simulink model "CS_ABS_KN_S"  (R2019a)
settings: Solver=ode45  StartTime=0  StopTime=10  FixedStep=0.002  RelTol=1e-6  AbsTol=1e-6
values from neighbouring files (symbols this model uses):
  AdCo = 0    [CS_ABS_KN.m]
  MoInRed = SloInRed/SloIn    (= 0.666666666667)    [CS_ABS_KN.m]
  RBP = 0.4    [CS_ABS_KN.m]
  SlMax = 0.15    [CS_ABS_KN.m]
  SloDe_ = SloDe/MBP    (= 3.33333333333)    [CS_ABS_KN.m]
  SloIn_ = SloIn/MBP    (= 10)    [CS_ABS_KN.m]
undefined symbols (not defined in the file or in its folder): DiscIntNeverNeededParam
libraries: Solver_SF x1
settings Model: ExtModeTrigMode=oneshot  ExtModeArmWhenConnect=off  Creator=Malan  LastModifiedBy=d001896
settings SolverCC: AutoScaleAbsTol=off  AlgebraicLoopSolver=LineSearch
settings DataIOCC: SaveFormat=Array  SignalLoggingSaveFormat=ModelDataLogs  ReturnWorkspaceOutputs=off  SignalLoggingName=sigsOut
settings OptimizationCC: BlockReduction=off  BooleanDataType=off  ExpressionDepthLimit=2147483647  InitFltsAndDblsToZero=on  LifeSpan=inf
settings DebuggingCC: AlgebraicLoopMsg=none  SaveWithParameterizedLinksMsg=none  UnderspecifiedInitializationDetection=Classic  MergeDetectMultiDrivingBlocksExec=none  SignalResolutionControl=TryResolveAllWithWarning  InheritedTsInSrcMsg=none  MultiTaskDSMMsg=warning  MultiTaskCondExecSysMsg=none  FcnCallInpInsideContextMsg=warning  StateNameClashWarn=warning  SFUnexpectedBacktrackingDiag=warning  SFNoUnconditionalDefaultTransitionDiag=warning  SFExecutionAtInitializationDiag=none  ArithmeticOperatorsInVariantConditions=warning
settings HardwareCC: ProdBitPerPointer=32  ProdBitPerSizeT=32  ProdBitPerPtrDiffT=32  ProdLargestAtomicFloat=None  ProdIntDivRoundTo=Undefined  ProdEndianess=Unspecified  ProdWordSize=32  ProdHWDeviceType=32-bit Generic  TargetUnknown=on
settings ModelReferenceCC: PropagateSignalLabelsOutOfModel=off
settings SFSimCC: SimUseLocalCustomCode=off
settings RTWCC: TemplateMakefile=grt_vc.tmf  RTWUseLocalCustomCode=off
settings CodeAppCC: StateflowObjectComments=on
settings GRTTargetCC: TargetFcnLib=ansi_tfl_tmw.mat  TargetLangStandard=C89/C90 (ANSI)  CombineOutputUpdateFcns=off  GRTInterface=on
settings ConfigComp: CovMetricSettings=dw  CovHtmlReporting=on  CovSaveCumulativeToWorkspaceVar=on  CovSaveSingleToWorkspaceVar=on  CovExternalEMLEnable=off

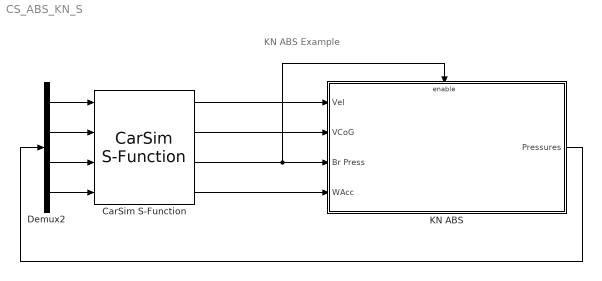
== system CS_ABS_KN_S ==
  note: KN ABS Example
  CarSim S-Function : Solver_SF/CarSim S-Function  Priority=1  SIMFILE=simfile.sim
  Demux2 : Demux
  KN ABS : Subsystem
  wires:
  CarSim S-Function/1 -> KN ABS/1(Vel)
  CarSim S-Function/2 -> KN ABS/2(VCoG)
  CarSim S-Function/3 -> KN ABS/Enable, KN ABS/3(Br Press)
  CarSim S-Function/4 -> KN ABS/4(WAcc)
  KN ABS/1(Pressures) -> Demux2/1
  Demux2/1 -> CarSim S-Function/1
  Demux2/2 -> CarSim S-Function/2
  Demux2/3 -> CarSim S-Function/3
  Demux2/4 -> CarSim S-Function/4

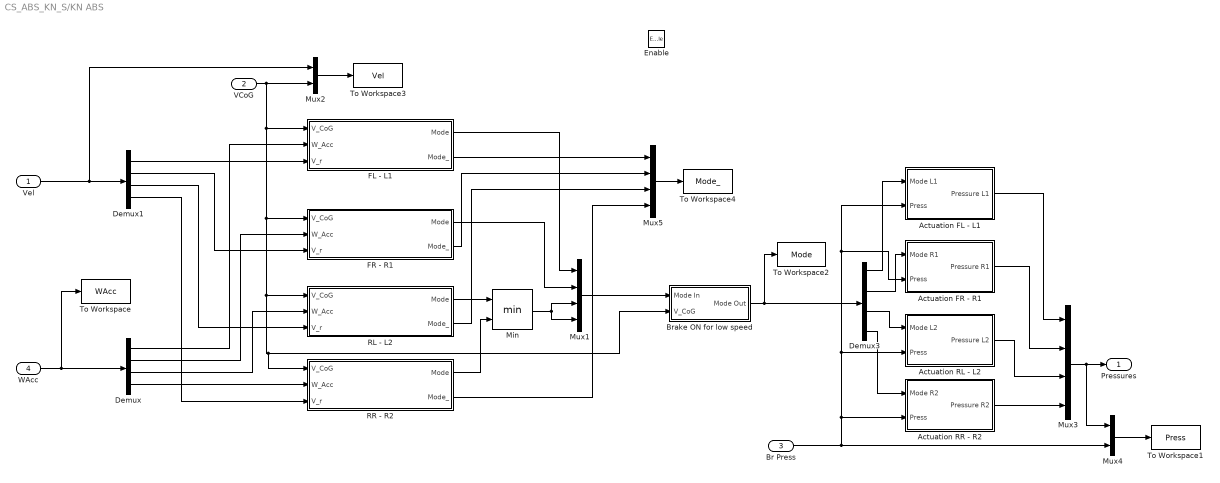
== system CS_ABS_KN_S/KN ABS ==
  Vel : Inport
  VCoG : Inport  Port=2
  Br Press : Inport  Port=3
  WAcc : Inport  Port=4
  Enable : EnablePort
  Actuation FL - L1 : Subsystem  TreatAsAtomicUnit=on
  Actuation FR - R1 : Subsystem  TreatAsAtomicUnit=on
  Actuation RL - L2 : Subsystem  TreatAsAtomicUnit=on
  Actuation RR - R2 : Subsystem  TreatAsAtomicUnit=on
  Brake ON for low speed : Subsystem  TreatAsAtomicUnit=on
  Demux : Demux
  Demux1 : Demux
  Demux3 : Demux
  FL - L1 : Subsystem  TreatAsAtomicUnit=on
  FR - R1 : Subsystem  TreatAsAtomicUnit=on
  Min : MinMax  Inputs=2  SaturateOnIntegerOverflow=on  InputSameDT=on
  Mux1 : Mux
  Mux2 : Mux  Inputs=2
  Mux3 : Mux
  Mux4 : Mux  Inputs=2
  Mux5 : Mux
  RL - L2 : Subsystem  TreatAsAtomicUnit=on
  RR - R2 : Subsystem  TreatAsAtomicUnit=on
  To Workspace : ToWorkspace  VariableName=WAcc  SaveFormat=Structure With Time  SampleTime=-1
  To Workspace1 : ToWorkspace  VariableName=Press  SaveFormat=Structure With Time  SampleTime=-1
  To Workspace2 : ToWorkspace  VariableName=Mode  SaveFormat=Structure With Time  SampleTime=-1
  To Workspace3 : ToWorkspace  VariableName=Vel  SaveFormat=Structure With Time  SampleTime=-1
  To Workspace4 : ToWorkspace  VariableName=Mode_  SaveFormat=Structure With Time  SampleTime=-1
  Pressures : Outport  InitialOutput=[0 0 0 0]
  wires:
  Mux3/1 -> Mux4/1, Pressures/1
  RL - L2/2(Mode_) -> Mux5/3
  RR - R2/2(Mode_) -> Mux5/4
  FL - L1/2(Mode_) -> Mux5/1
  FR - R1/2(Mode_) -> Mux5/2
  Demux/2 -> FR - R1/2(W_Acc)
  FL - L1/1(Mode) -> Mux1/1
  Demux3/1 -> Actuation FL - L1/1(Mode L1)
  Demux3/3 -> Actuation RL - L2/1(Mode L2)
  VCoG/1 -> Brake ON for low speed/2(V_CoG), RR - R2/1(V_CoG), RL - L2/1(V_CoG), FR - R1/1(V_CoG), FL - L1/1(V_CoG), Mux2/2
  Demux/3 -> RL - L2/2(W_Acc)
  Demux1/2 -> FR - R1/3(V_r)
  Demux/1 -> FL - L1/2(W_Acc)
  Brake ON for low speed/1(Mode Out) -> To Workspace2/1, Demux3/1
  Br Press/1 -> Actuation RR - R2/2(Press), Actuation RL - L2/2(Press), Actuation FR - R1/2(Press), Actuation FL - L1/2(Press), Mux4/2
  Demux1/3 -> RL - L2/3(V_r)
  Demux1/4 -> RR - R2/3(V_r)
  Vel/1 -> Mux2/1, Demux1/1
  Mux1/1 -> Brake ON for low speed/1(Mode In)
  Actuation RL - L2/1(Pressure L2) -> Mux3/3
  Actuation RR - R2/1(Pressure R2) -> Mux3/4
  Actuation FR - R1/1(Pressure R1) -> Mux3/2
  WAcc/1 -> To Workspace/1, Demux/1
  Demux3/2 -> Actuation FR - R1/1(Mode R1)
  Demux1/1 -> FL - L1/3(V_r)
  Mux2/1 -> To Workspace3/1
  Min/1 -> Mux1/4, Mux1/3
  Demux/4 -> RR - R2/2(W_Acc)
  FR - R1/1(Mode) -> Mux1/2
  Mux4/1 -> To Workspace1/1
  RR - R2/1(Mode) -> Min/2
  Demux3/4 -> Actuation RR - R2/1(Mode R2)
  RL - L2/1(Mode) -> Min/1
  Mux5/1 -> To Workspace4/1
  Actuation FL - L1/1(Pressure L1) -> Mux3/1

== system CS_ABS_KN_S/KN ABS/Actuation FL - L1 ==
  Mode L1 : Inport
  Press : Inport  Port=2
  Discrete-Time Integrator2 : DiscreteIntegrator  IntegratorMethod=Integration: Backward Euler  gainval=1  SampleTime=-1  LimitOutput=on  UpperSaturationLimit=1  LowerSaturationLimit=0  ICPrevOutput=DiscIntNeverNeededParam  ICPrevScaledInput=DiscIntNeverNeededParam
  If : If
  If Action Subsystem : Subsystem  TreatAsAtomicUnit=on
  If Action Subsystem1 : Subsystem  TreatAsAtomicUnit=on
  Merge : Merge
  Product : Product
  Pressure L1 : Outport
  wires:
  If/2 -> If Action Subsystem/Action
  If Action Subsystem/1(Out1) -> Merge/2
  If/1 -> If Action Subsystem1/Action
  If Action Subsystem1/1(Out1) -> Merge/1
  Merge/1 -> Discrete-Time Integrator2/1
  Mode L1/1 -> If Action Subsystem1/1(In1), If Action Subsystem/1(In1), If/1
  Discrete-Time Integrator2/1 -> Product/1
  Product/1 -> Pressure L1/1
  Press/1 -> Product/2

== system CS_ABS_KN_S/KN ABS/Actuation FR - R1 ==
  Mode R1 : Inport
  Press : Inport  Port=2
  Discrete-Time Integrator2 : DiscreteIntegrator  IntegratorMethod=Integration: Backward Euler  gainval=1  SampleTime=-1  LimitOutput=on  UpperSaturationLimit=1  LowerSaturationLimit=0  ICPrevOutput=DiscIntNeverNeededParam  ICPrevScaledInput=DiscIntNeverNeededParam
  If : If
  If Action Subsystem : Subsystem  TreatAsAtomicUnit=on
  If Action Subsystem1 : Subsystem  TreatAsAtomicUnit=on
  Merge : Merge
  Product : Product
  Pressure R1 : Outport
  wires:
  If/2 -> If Action Subsystem/Action
  If Action Subsystem/1(Out1) -> Merge/2
  If/1 -> If Action Subsystem1/Action
  If Action Subsystem1/1(Out1) -> Merge/1
  Merge/1 -> Discrete-Time Integrator2/1
  Mode R1/1 -> If Action Subsystem1/1(In1), If Action Subsystem/1(In1), If/1
  Press/1 -> Product/2
  Discrete-Time Integrator2/1 -> Product/1
  Product/1 -> Pressure R1/1

== system CS_ABS_KN_S/KN ABS/Actuation RL - L2 ==
  Mode L2 : Inport
  Press : Inport  Port=2
  Discrete-Time Integrator2 : DiscreteIntegrator  IntegratorMethod=Integration: Backward Euler  gainval=1  SampleTime=-1  LimitOutput=on  UpperSaturationLimit=1  LowerSaturationLimit=0  ICPrevOutput=DiscIntNeverNeededParam  ICPrevScaledInput=DiscIntNeverNeededParam
  Gain : Gain  Gain=RBP
  If : If
  If Action Subsystem : Subsystem  TreatAsAtomicUnit=on
  If Action Subsystem1 : Subsystem  TreatAsAtomicUnit=on
  Merge : Merge
  Product : Product
  Pressure L2 : Outport
  wires:
  If/2 -> If Action Subsystem/Action
  If Action Subsystem/1(Out1) -> Merge/2
  If/1 -> If Action Subsystem1/Action
  If Action Subsystem1/1(Out1) -> Merge/1
  Merge/1 -> Discrete-Time Integrator2/1
  Discrete-Time Integrator2/1 -> Gain/1
  Mode L2/1 -> If Action Subsystem1/1(In1), If Action Subsystem/1(In1), If/1
  Press/1 -> Product/2
  Gain/1 -> Product/1
  Product/1 -> Pressure L2/1

== system CS_ABS_KN_S/KN ABS/Actuation RR - R2 ==
  Mode R2 : Inport
  Press : Inport  Port=2
  Discrete-Time Integrator2 : DiscreteIntegrator  IntegratorMethod=Integration: Backward Euler  gainval=1  SampleTime=-1  LimitOutput=on  UpperSaturationLimit=1  LowerSaturationLimit=0  ICPrevOutput=DiscIntNeverNeededParam  ICPrevScaledInput=DiscIntNeverNeededParam
  Gain : Gain  Gain=RBP
  If : If
  If Action Subsystem : Subsystem  TreatAsAtomicUnit=on
  If Action Subsystem1 : Subsystem  TreatAsAtomicUnit=on
  Merge : Merge
  Product : Product
  Pressure R2 : Outport
  wires:
  Discrete-Time Integrator2/1 -> Gain/1
  If/2 -> If Action Subsystem/Action
  If Action Subsystem/1(Out1) -> Merge/2
  If/1 -> If Action Subsystem1/Action
  If Action Subsystem1/1(Out1) -> Merge/1
  Merge/1 -> Discrete-Time Integrator2/1
  Mode R2/1 -> If Action Subsystem1/1(In1), If Action Subsystem/1(In1), If/1
  Press/1 -> Product/2
  Gain/1 -> Product/1
  Product/1 -> Pressure R2/1

== system CS_ABS_KN_S/KN ABS/Brake ON for low speed ==
  Mode In : Inport
  V_CoG : Inport  Port=2
  If : If  IfExpression=u1 >= Vmin
  If Action Subsystem : Subsystem  TreatAsAtomicUnit=on
  If Action Subsystem1 : Subsystem  TreatAsAtomicUnit=on
  Merge : Merge
  "[1 1 1 1]" : Constant  Value=[1 1 1 1]
  Mode Out : Outport
  wires:
  "[1 1 1 1]"/1 -> If Action Subsystem/1(In1)
  V_CoG/1 -> If/1
  Mode In/1 -> If Action Subsystem1/1(In1)
  If/2 -> If Action Subsystem/Action
  If Action Subsystem/1(Out1) -> Merge/2
  If/1 -> If Action Subsystem1/Action
  If Action Subsystem1/1(Out1) -> Merge/1
  Merge/1 -> Mode Out/1

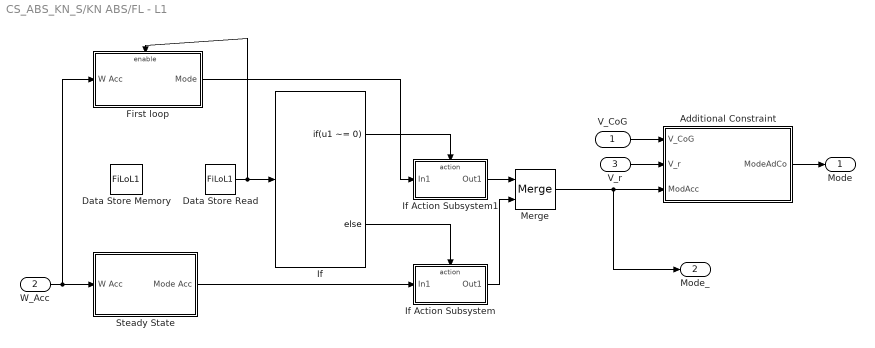
== system CS_ABS_KN_S/KN ABS/FL - L1 ==
  V_CoG : Inport
  W_Acc : Inport  Port=2
  V_r : Inport  Port=3
  Additional Constraint : Subsystem
  Data Store Memory : DataStoreMemory  DataStoreName=FiLoL1  InitialValue=1  ShowAdditionalParam=off
  Data Store Read : DataStoreRead  DataStoreName=FiLoL1
  First loop : Subsystem
  If : If  IfExpression=u1 ~= 0
  If Action Subsystem : Subsystem  TreatAsAtomicUnit=on
  If Action Subsystem1 : Subsystem  TreatAsAtomicUnit=on
  Merge : Merge
  Steady State : Subsystem
  Mode : Outport
  Mode_ : Outport  Port=2
  wires:
  V_CoG/1 -> Additional Constraint/1(V_CoG)
  V_r/1 -> Additional Constraint/2("V_r ")
  W_Acc/1 -> Steady State/1(W Acc), First loop/1(W Acc)
  Data Store Read/1 -> If/1, First loop/Enable
  First loop/1(Mode) -> If Action Subsystem1/1(In1)
  Steady State/1(Mode Acc) -> If Action Subsystem/1(In1)
  If/1 -> If Action Subsystem1/Action
  If/2 -> If Action Subsystem/Action
  If Action Subsystem1/1(Out1) -> Merge/1
  If Action Subsystem/1(Out1) -> Merge/2
  Merge/1 -> Mode_/1, Additional Constraint/3(ModAcc)
  Additional Constraint/1(ModeAdCo) -> Mode/1

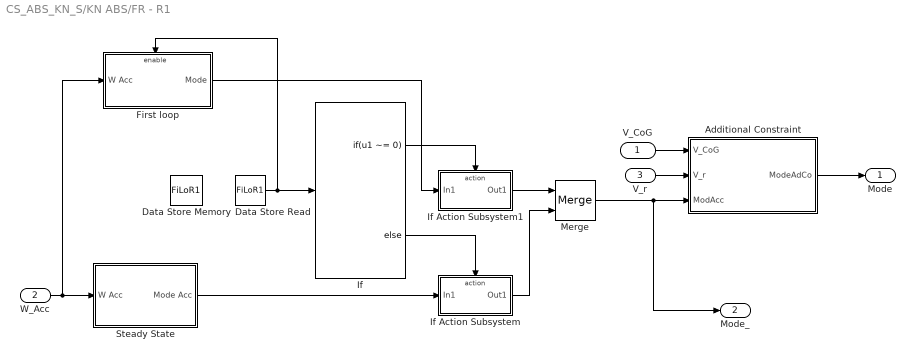
== system CS_ABS_KN_S/KN ABS/FR - R1 ==
  V_CoG : Inport
  W_Acc : Inport  Port=2
  V_r : Inport  Port=3
  Additional Constraint : Subsystem
  Data Store Memory : DataStoreMemory  DataStoreName=FiLoR1  InitialValue=1  ShowAdditionalParam=off
  Data Store Read : DataStoreRead  DataStoreName=FiLoR1
  First loop : Subsystem
  If : If  IfExpression=u1 ~= 0
  If Action Subsystem : Subsystem  TreatAsAtomicUnit=on
  If Action Subsystem1 : Subsystem  TreatAsAtomicUnit=on
  Merge : Merge
  Steady State : Subsystem
  Mode : Outport
  Mode_ : Outport  Port=2
  wires:
  V_CoG/1 -> Additional Constraint/1(V_CoG)
  V_r/1 -> Additional Constraint/2("V_r ")
  W_Acc/1 -> Steady State/1(W Acc), First loop/1(W Acc)
  Data Store Read/1 -> First loop/Enable, If/1
  Steady State/1(Mode Acc) -> If Action Subsystem/1(In1)
  First loop/1(Mode) -> If Action Subsystem1/1(In1)
  If/1 -> If Action Subsystem1/Action
  If/2 -> If Action Subsystem/Action
  If Action Subsystem1/1(Out1) -> Merge/1
  If Action Subsystem/1(Out1) -> Merge/2
  Additional Constraint/1(ModeAdCo) -> Mode/1
  Merge/1 -> Mode_/1, Additional Constraint/3(ModAcc)

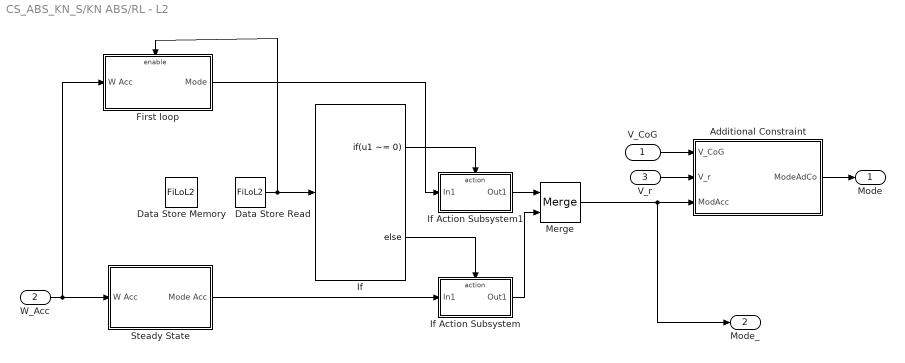
== system CS_ABS_KN_S/KN ABS/RL - L2 ==
  V_CoG : Inport
  W_Acc : Inport  Port=2
  V_r : Inport  Port=3
  Additional Constraint : Subsystem
  Data Store Memory : DataStoreMemory  DataStoreName=FiLoL2  InitialValue=1  ShowAdditionalParam=off
  Data Store Read : DataStoreRead  DataStoreName=FiLoL2
  First loop : Subsystem
  If : If  IfExpression=u1 ~= 0
  If Action Subsystem : Subsystem  TreatAsAtomicUnit=on
  If Action Subsystem1 : Subsystem  TreatAsAtomicUnit=on
  Merge : Merge
  Steady State : Subsystem
  Mode : Outport
  Mode_ : Outport  Port=2
  wires:
  V_CoG/1 -> Additional Constraint/1(V_CoG)
  V_r/1 -> Additional Constraint/2("V_r ")
  W_Acc/1 -> Steady State/1(W Acc), First loop/1(W Acc)
  Data Store Read/1 -> If/1, First loop/Enable
  Steady State/1(Mode Acc) -> If Action Subsystem/1(In1)
  First loop/1(Mode) -> If Action Subsystem1/1(In1)
  If/1 -> If Action Subsystem1/Action
  If/2 -> If Action Subsystem/Action
  If Action Subsystem1/1(Out1) -> Merge/1
  If Action Subsystem/1(Out1) -> Merge/2
  Additional Constraint/1(ModeAdCo) -> Mode/1
  Merge/1 -> Mode_/1, Additional Constraint/3(ModAcc)

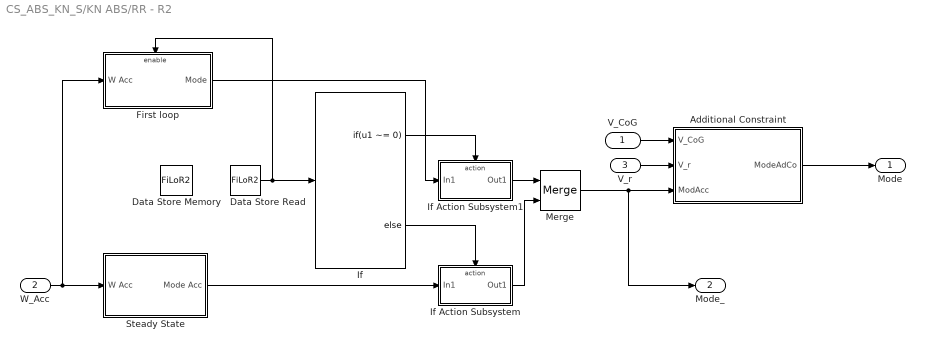
== system CS_ABS_KN_S/KN ABS/RR - R2 ==
  V_CoG : Inport
  W_Acc : Inport  Port=2
  V_r : Inport  Port=3
  Additional Constraint : Subsystem
  Data Store Memory : DataStoreMemory  DataStoreName=FiLoR2  InitialValue=1  ShowAdditionalParam=off
  Data Store Read : DataStoreRead  DataStoreName=FiLoR2
  First loop : Subsystem
  If : If  IfExpression=u1 ~= 0
  If Action Subsystem : Subsystem  TreatAsAtomicUnit=on
  If Action Subsystem1 : Subsystem  TreatAsAtomicUnit=on
  Merge : Merge
  Steady State : Subsystem
  Mode : Outport
  Mode_ : Outport  Port=2
  wires:
  V_CoG/1 -> Additional Constraint/1(V_CoG)
  V_r/1 -> Additional Constraint/2("V_r ")
  W_Acc/1 -> Steady State/1(W Acc), First loop/1(W Acc)
  Data Store Read/1 -> First loop/Enable, If/1
  Steady State/1(Mode Acc) -> If Action Subsystem/1(In1)
  First loop/1(Mode) -> If Action Subsystem1/1(In1)
  If/1 -> If Action Subsystem1/Action
  If/2 -> If Action Subsystem/Action
  If Action Subsystem1/1(Out1) -> Merge/1
  If Action Subsystem/1(Out1) -> Merge/2
  Additional Constraint/1(ModeAdCo) -> Mode/1
  Merge/1 -> Mode_/1, Additional Constraint/3(ModAcc)

== system CS_ABS_KN_S/KN ABS/Actuation FL - L1/If Action Subsystem ==
  In1 : Inport
  Action Port : ActionPort  ActionPortLabel=else
  Gain1 : Gain  Gain=SloDe_
  Out1 : Outport
  wires:
  In1/1 -> Gain1/1
  Gain1/1 -> Out1/1

== system CS_ABS_KN_S/KN ABS/Actuation FL - L1/If Action Subsystem1 ==
  In1 : Inport
  Action Port : ActionPort  ActionPortLabel=if(u1 > 0)
  Gain : Gain  Gain=SloIn_
  Out1 : Outport
  wires:
  In1/1 -> Gain/1
  Gain/1 -> Out1/1

== system CS_ABS_KN_S/KN ABS/Actuation FR - R1/If Action Subsystem ==
  In1 : Inport
  Action Port : ActionPort  ActionPortLabel=else
  Gain1 : Gain  Gain=SloDe_
  Out1 : Outport
  wires:
  In1/1 -> Gain1/1
  Gain1/1 -> Out1/1

== system CS_ABS_KN_S/KN ABS/Actuation FR - R1/If Action Subsystem1 ==
  In1 : Inport
  Action Port : ActionPort  ActionPortLabel=if(u1 > 0)
  Gain : Gain  Gain=SloIn_
  Out1 : Outport
  wires:
  In1/1 -> Gain/1
  Gain/1 -> Out1/1

== system CS_ABS_KN_S/KN ABS/Actuation RL - L2/If Action Subsystem ==
  In1 : Inport
  Action Port : ActionPort  ActionPortLabel=else
  Gain1 : Gain  Gain=SloDe_
  Out1 : Outport
  wires:
  In1/1 -> Gain1/1
  Gain1/1 -> Out1/1

== system CS_ABS_KN_S/KN ABS/Actuation RL - L2/If Action Subsystem1 ==
  In1 : Inport
  Action Port : ActionPort  ActionPortLabel=if(u1 > 0)
  Gain : Gain  Gain=SloIn_
  Out1 : Outport
  wires:
  In1/1 -> Gain/1
  Gain/1 -> Out1/1

== system CS_ABS_KN_S/KN ABS/Actuation RR - R2/If Action Subsystem ==
  In1 : Inport
  Action Port : ActionPort  ActionPortLabel=else
  Gain1 : Gain  Gain=SloDe_
  Out1 : Outport
  wires:
  In1/1 -> Gain1/1
  Gain1/1 -> Out1/1

== system CS_ABS_KN_S/KN ABS/Actuation RR - R2/If Action Subsystem1 ==
  In1 : Inport
  Action Port : ActionPort  ActionPortLabel=if(u1 > 0)
  Gain : Gain  Gain=SloIn_
  Out1 : Outport
  wires:
  In1/1 -> Gain/1
  Gain/1 -> Out1/1

== system CS_ABS_KN_S/KN ABS/Brake ON for low speed/If Action Subsystem ==
  In1 : Inport
  Action Port : ActionPort  ActionPortLabel=else
  Out1 : Outport
  wires:
  In1/1 -> Out1/1

== system CS_ABS_KN_S/KN ABS/Brake ON for low speed/If Action Subsystem1 ==
  In1 : Inport
  Action Port : ActionPort  ActionPortLabel=if(u1 >= Vmin)
  Out1 : Outport
  wires:
  In1/1 -> Out1/1

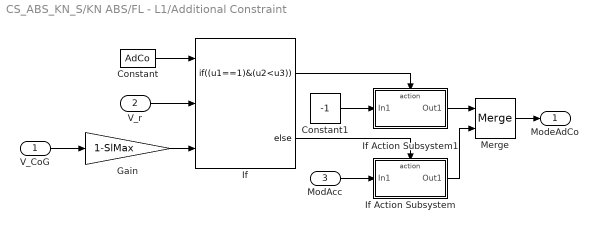
== system CS_ABS_KN_S/KN ABS/FL - L1/Additional Constraint ==
  V_CoG : Inport
  "V_r " : Inport  Port=2
  ModAcc : Inport  Port=3
  Constant : Constant  Value=AdCo
  Constant1 : Constant  Value=-1
  Gain : Gain  Gain=1-SlMax
  If : If  NumInputs=3  IfExpression=(u1==1)&(u2<u3)
  If Action Subsystem : Subsystem  TreatAsAtomicUnit=on
  If Action Subsystem1 : Subsystem  TreatAsAtomicUnit=on
  Merge : Merge
  ModeAdCo : Outport
  wires:
  Gain/1 -> If/3
  V_CoG/1 -> Gain/1
  "V_r "/1 -> If/2
  Merge/1 -> ModeAdCo/1
  ModAcc/1 -> If Action Subsystem/1(In1)
  If/2 -> If Action Subsystem/Action
  If Action Subsystem/1(Out1) -> Merge/2
  If/1 -> If Action Subsystem1/Action
  If Action Subsystem1/1(Out1) -> Merge/1
  Constant/1 -> If/1
  Constant1/1 -> If Action Subsystem1/1(In1)

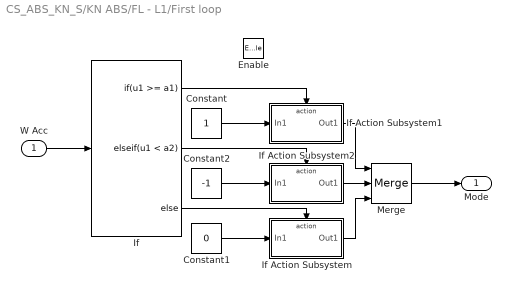
== system CS_ABS_KN_S/KN ABS/FL - L1/First loop ==
  W Acc : Inport
  Enable : EnablePort
  Constant : Constant
  Constant1 : Constant  Value=0
  Constant2 : Constant  Value=-1
  If : If  IfExpression=u1 >= a1  ElseIfExpressions=u1 < a2
  If Action Subsystem : Subsystem  TreatAsAtomicUnit=on
  If Action Subsystem1 : Subsystem  TreatAsAtomicUnit=on
  If Action Subsystem2 : Subsystem  TreatAsAtomicUnit=on
  Merge : Merge  Inputs=3
  Mode : Outport
  wires:
  Constant2/1 -> If Action Subsystem2/1(In1)
  If/3 -> If Action Subsystem/Action
  If/1 -> If Action Subsystem1/Action
  If Action Subsystem1/1(Out1) -> Merge/1
  If/2 -> If Action Subsystem2/Action
  If Action Subsystem2/1(Out1) -> Merge/2
  If Action Subsystem/1(Out1) -> Merge/3
  W Acc/1 -> If/1
  Merge/1 -> Mode/1
  Constant1/1 -> If Action Subsystem/1(In1)
  Constant/1 -> If Action Subsystem1/1(In1)

== system CS_ABS_KN_S/KN ABS/FL - L1/If Action Subsystem ==
  In1 : Inport
  Action Port : ActionPort  ActionPortLabel=else
  Out1 : Outport
  wires:
  In1/1 -> Out1/1

== system CS_ABS_KN_S/KN ABS/FL - L1/If Action Subsystem1 ==
  In1 : Inport
  Action Port : ActionPort  ActionPortLabel=if(u1 ~= 0)
  Out1 : Outport
  wires:
  In1/1 -> Out1/1

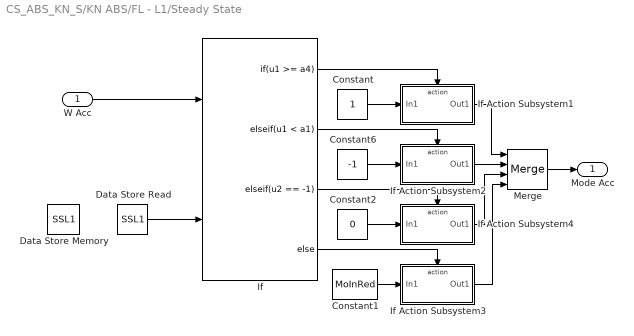
== system CS_ABS_KN_S/KN ABS/FL - L1/Steady State ==
  W Acc : Inport
  Constant : Constant
  Constant1 : Constant  Value=MoInRed
  Constant2 : Constant  Value=0
  Constant6 : Constant  Value=-1
  Data Store Memory : DataStoreMemory  DataStoreName=SSL1  InitialValue=-1  ShowAdditionalParam=off
  Data Store Read : DataStoreRead  DataStoreName=SSL1
  If : If  NumInputs=2  IfExpression=u1 >= a4  ElseIfExpressions=u1 < a1, u2 == -1
  If Action Subsystem1 : Subsystem  TreatAsAtomicUnit=on
  If Action Subsystem2 : Subsystem  TreatAsAtomicUnit=on
  If Action Subsystem3 : Subsystem  TreatAsAtomicUnit=on
  If Action Subsystem4 : Subsystem  TreatAsAtomicUnit=on
  Merge : Merge  Inputs=4
  Mode Acc : Outport
  wires:
  Data Store Read/1 -> If/2
  Constant2/1 -> If Action Subsystem4/1(In1)
  Constant1/1 -> If Action Subsystem3/1(In1)
  W Acc/1 -> If/1
  Merge/1 -> Mode Acc/1
  Constant6/1 -> If Action Subsystem2/1(In1)
  If/4 -> If Action Subsystem3/Action
  If/1 -> If Action Subsystem1/Action
  If Action Subsystem1/1(Out1) -> Merge/1
  If/2 -> If Action Subsystem2/Action
  If Action Subsystem2/1(Out1) -> Merge/2
  Constant/1 -> If Action Subsystem1/1(In1)
  If Action Subsystem4/1(Out1) -> Merge/3
  If Action Subsystem3/1(Out1) -> Merge/4
  If/3 -> If Action Subsystem4/Action

== system CS_ABS_KN_S/KN ABS/FR - R1/Additional Constraint ==
  V_CoG : Inport
  "V_r " : Inport  Port=2
  ModAcc : Inport  Port=3
  Constant : Constant  Value=AdCo
  Constant1 : Constant  Value=-1
  Gain : Gain  Gain=1-SlMax
  If : If  NumInputs=3  IfExpression=(u1==1)&(u2<u3)
  If Action Subsystem : Subsystem  TreatAsAtomicUnit=on
  If Action Subsystem1 : Subsystem  TreatAsAtomicUnit=on
  Merge : Merge
  ModeAdCo : Outport
  wires:
  Gain/1 -> If/3
  V_CoG/1 -> Gain/1
  "V_r "/1 -> If/2
  Merge/1 -> ModeAdCo/1
  ModAcc/1 -> If Action Subsystem/1(In1)
  If/2 -> If Action Subsystem/Action
  If Action Subsystem/1(Out1) -> Merge/2
  If/1 -> If Action Subsystem1/Action
  If Action Subsystem1/1(Out1) -> Merge/1
  Constant/1 -> If/1
  Constant1/1 -> If Action Subsystem1/1(In1)

== system CS_ABS_KN_S/KN ABS/FR - R1/First loop ==
  W Acc : Inport
  Enable : EnablePort
  Constant : Constant
  Constant1 : Constant  Value=0
  Constant2 : Constant  Value=-1
  If : If  IfExpression=u1 >= a1  ElseIfExpressions=u1 < a2
  If Action Subsystem : Subsystem  TreatAsAtomicUnit=on
  If Action Subsystem1 : Subsystem  TreatAsAtomicUnit=on
  If Action Subsystem2 : Subsystem  TreatAsAtomicUnit=on
  Merge : Merge  Inputs=3
  Mode : Outport
  wires:
  Constant2/1 -> If Action Subsystem2/1(In1)
  If/3 -> If Action Subsystem/Action
  If/1 -> If Action Subsystem1/Action
  If Action Subsystem1/1(Out1) -> Merge/1
  If/2 -> If Action Subsystem2/Action
  If Action Subsystem2/1(Out1) -> Merge/2
  If Action Subsystem/1(Out1) -> Merge/3
  W Acc/1 -> If/1
  Merge/1 -> Mode/1
  Constant1/1 -> If Action Subsystem/1(In1)
  Constant/1 -> If Action Subsystem1/1(In1)

== system CS_ABS_KN_S/KN ABS/FR - R1/If Action Subsystem ==
  In1 : Inport
  Action Port : ActionPort  ActionPortLabel=else
  Out1 : Outport
  wires:
  In1/1 -> Out1/1

== system CS_ABS_KN_S/KN ABS/FR - R1/If Action Subsystem1 ==
  In1 : Inport
  Action Port : ActionPort  ActionPortLabel=if(u1 ~= 0)
  Out1 : Outport
  wires:
  In1/1 -> Out1/1

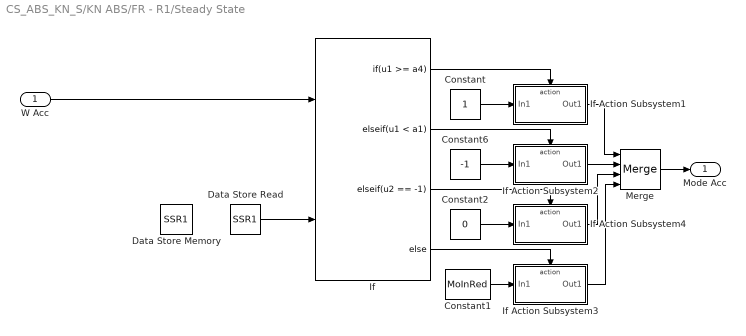
== system CS_ABS_KN_S/KN ABS/FR - R1/Steady State ==
  W Acc : Inport
  Constant : Constant
  Constant1 : Constant  Value=MoInRed
  Constant2 : Constant  Value=0
  Constant6 : Constant  Value=-1
  Data Store Memory : DataStoreMemory  DataStoreName=SSR1  InitialValue=-1  ShowAdditionalParam=off
  Data Store Read : DataStoreRead  DataStoreName=SSR1
  If : If  NumInputs=2  IfExpression=u1 >= a4  ElseIfExpressions=u1 < a1, u2 == -1
  If Action Subsystem1 : Subsystem  TreatAsAtomicUnit=on
  If Action Subsystem2 : Subsystem  TreatAsAtomicUnit=on
  If Action Subsystem3 : Subsystem  TreatAsAtomicUnit=on
  If Action Subsystem4 : Subsystem  TreatAsAtomicUnit=on
  Merge : Merge  Inputs=4
  Mode Acc : Outport
  wires:
  Data Store Read/1 -> If/2
  Constant2/1 -> If Action Subsystem4/1(In1)
  Constant1/1 -> If Action Subsystem3/1(In1)
  W Acc/1 -> If/1
  Merge/1 -> Mode Acc/1
  Constant6/1 -> If Action Subsystem2/1(In1)
  If/4 -> If Action Subsystem3/Action
  If/1 -> If Action Subsystem1/Action
  If Action Subsystem1/1(Out1) -> Merge/1
  If/2 -> If Action Subsystem2/Action
  If Action Subsystem2/1(Out1) -> Merge/2
  Constant/1 -> If Action Subsystem1/1(In1)
  If Action Subsystem4/1(Out1) -> Merge/3
  If Action Subsystem3/1(Out1) -> Merge/4
  If/3 -> If Action Subsystem4/Action

== system CS_ABS_KN_S/KN ABS/RL - L2/Additional Constraint ==
  V_CoG : Inport
  "V_r " : Inport  Port=2
  ModAcc : Inport  Port=3
  Constant : Constant  Value=AdCo
  Constant1 : Constant  Value=-1
  Gain : Gain  Gain=1-SlMax
  If : If  NumInputs=3  IfExpression=(u1==1)&(u2<u3)
  If Action Subsystem : Subsystem  TreatAsAtomicUnit=on
  If Action Subsystem1 : Subsystem  TreatAsAtomicUnit=on
  Merge : Merge
  ModeAdCo : Outport
  wires:
  Gain/1 -> If/3
  V_CoG/1 -> Gain/1
  "V_r "/1 -> If/2
  Merge/1 -> ModeAdCo/1
  ModAcc/1 -> If Action Subsystem/1(In1)
  If/2 -> If Action Subsystem/Action
  If Action Subsystem/1(Out1) -> Merge/2
  If/1 -> If Action Subsystem1/Action
  If Action Subsystem1/1(Out1) -> Merge/1
  Constant/1 -> If/1
  Constant1/1 -> If Action Subsystem1/1(In1)

== system CS_ABS_KN_S/KN ABS/RL - L2/First loop ==
  W Acc : Inport
  Enable : EnablePort
  Constant : Constant
  Constant1 : Constant  Value=0
  Constant2 : Constant  Value=-1
  If : If  IfExpression=u1 >= a1  ElseIfExpressions=u1 < a2
  If Action Subsystem : Subsystem  TreatAsAtomicUnit=on
  If Action Subsystem1 : Subsystem  TreatAsAtomicUnit=on
  If Action Subsystem2 : Subsystem  TreatAsAtomicUnit=on
  Merge : Merge  Inputs=3
  Mode : Outport
  wires:
  Constant2/1 -> If Action Subsystem2/1(In1)
  If/3 -> If Action Subsystem/Action
  If/1 -> If Action Subsystem1/Action
  If Action Subsystem1/1(Out1) -> Merge/1
  If/2 -> If Action Subsystem2/Action
  If Action Subsystem2/1(Out1) -> Merge/2
  If Action Subsystem/1(Out1) -> Merge/3
  W Acc/1 -> If/1
  Merge/1 -> Mode/1
  Constant1/1 -> If Action Subsystem/1(In1)
  Constant/1 -> If Action Subsystem1/1(In1)

== system CS_ABS_KN_S/KN ABS/RL - L2/If Action Subsystem ==
  In1 : Inport
  Action Port : ActionPort  ActionPortLabel=else
  Out1 : Outport
  wires:
  In1/1 -> Out1/1

== system CS_ABS_KN_S/KN ABS/RL - L2/If Action Subsystem1 ==
  In1 : Inport
  Action Port : ActionPort  ActionPortLabel=if(u1 ~= 0)
  Out1 : Outport
  wires:
  In1/1 -> Out1/1

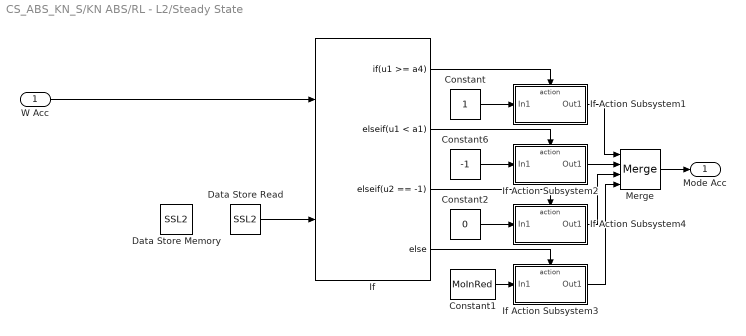
== system CS_ABS_KN_S/KN ABS/RL - L2/Steady State ==
  W Acc : Inport
  Constant : Constant
  Constant1 : Constant  Value=MoInRed
  Constant2 : Constant  Value=0
  Constant6 : Constant  Value=-1
  Data Store Memory : DataStoreMemory  DataStoreName=SSL2  InitialValue=-1  ShowAdditionalParam=off
  Data Store Read : DataStoreRead  DataStoreName=SSL2
  If : If  NumInputs=2  IfExpression=u1 >= a4  ElseIfExpressions=u1 < a1, u2 == -1
  If Action Subsystem1 : Subsystem  TreatAsAtomicUnit=on
  If Action Subsystem2 : Subsystem  TreatAsAtomicUnit=on
  If Action Subsystem3 : Subsystem  TreatAsAtomicUnit=on
  If Action Subsystem4 : Subsystem  TreatAsAtomicUnit=on
  Merge : Merge  Inputs=4
  Mode Acc : Outport
  wires:
  Data Store Read/1 -> If/2
  Constant2/1 -> If Action Subsystem4/1(In1)
  Constant1/1 -> If Action Subsystem3/1(In1)
  W Acc/1 -> If/1
  Merge/1 -> Mode Acc/1
  Constant6/1 -> If Action Subsystem2/1(In1)
  If/4 -> If Action Subsystem3/Action
  If/1 -> If Action Subsystem1/Action
  If Action Subsystem1/1(Out1) -> Merge/1
  If/2 -> If Action Subsystem2/Action
  If Action Subsystem2/1(Out1) -> Merge/2
  Constant/1 -> If Action Subsystem1/1(In1)
  If Action Subsystem4/1(Out1) -> Merge/3
  If Action Subsystem3/1(Out1) -> Merge/4
  If/3 -> If Action Subsystem4/Action

== system CS_ABS_KN_S/KN ABS/RR - R2/Additional Constraint ==
  V_CoG : Inport
  "V_r " : Inport  Port=2
  ModAcc : Inport  Port=3
  Constant : Constant  Value=AdCo
  Constant1 : Constant  Value=-1
  Gain : Gain  Gain=1-SlMax
  If : If  NumInputs=3  IfExpression=(u1==1)&(u2<u3)
  If Action Subsystem : Subsystem  TreatAsAtomicUnit=on
  If Action Subsystem1 : Subsystem  TreatAsAtomicUnit=on
  Merge : Merge
  ModeAdCo : Outport
  wires:
  Gain/1 -> If/3
  V_CoG/1 -> Gain/1
  "V_r "/1 -> If/2
  Merge/1 -> ModeAdCo/1
  ModAcc/1 -> If Action Subsystem/1(In1)
  If/2 -> If Action Subsystem/Action
  If Action Subsystem/1(Out1) -> Merge/2
  If/1 -> If Action Subsystem1/Action
  Constant/1 -> If/1
  Constant1/1 -> If Action Subsystem1/1(In1)
  If Action Subsystem1/1(Out1) -> Merge/1

== system CS_ABS_KN_S/KN ABS/RR - R2/First loop ==
  W Acc : Inport
  Enable : EnablePort
  Constant : Constant
  Constant1 : Constant  Value=0
  Constant2 : Constant  Value=-1
  If : If  IfExpression=u1 >= a1  ElseIfExpressions=u1 < a2
  If Action Subsystem : Subsystem  TreatAsAtomicUnit=on
  If Action Subsystem1 : Subsystem  TreatAsAtomicUnit=on
  If Action Subsystem2 : Subsystem  TreatAsAtomicUnit=on
  Merge : Merge  Inputs=3
  Mode : Outport
  wires:
  Constant2/1 -> If Action Subsystem2/1(In1)
  If/3 -> If Action Subsystem/Action
  If/1 -> If Action Subsystem1/Action
  If Action Subsystem1/1(Out1) -> Merge/1
  If/2 -> If Action Subsystem2/Action
  If Action Subsystem2/1(Out1) -> Merge/2
  If Action Subsystem/1(Out1) -> Merge/3
  W Acc/1 -> If/1
  Merge/1 -> Mode/1
  Constant1/1 -> If Action Subsystem/1(In1)
  Constant/1 -> If Action Subsystem1/1(In1)

== system CS_ABS_KN_S/KN ABS/RR - R2/If Action Subsystem ==
  In1 : Inport
  Action Port : ActionPort  ActionPortLabel=else
  Out1 : Outport
  wires:
  In1/1 -> Out1/1

== system CS_ABS_KN_S/KN ABS/RR - R2/If Action Subsystem1 ==
  In1 : Inport
  Action Port : ActionPort  ActionPortLabel=if(u1 ~= 0)
  Out1 : Outport
  wires:
  In1/1 -> Out1/1

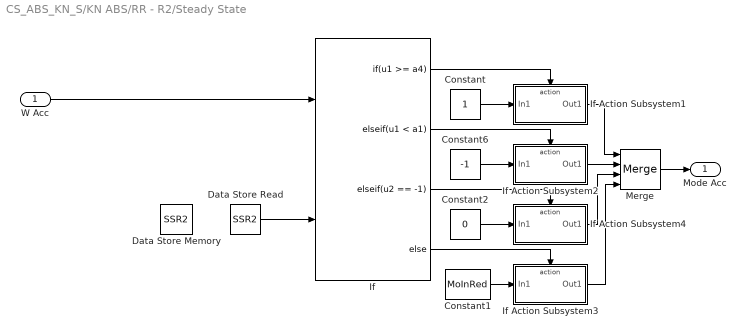
== system CS_ABS_KN_S/KN ABS/RR - R2/Steady State ==
  W Acc : Inport
  Constant : Constant
  Constant1 : Constant  Value=MoInRed
  Constant2 : Constant  Value=0
  Constant6 : Constant  Value=-1
  Data Store Memory : DataStoreMemory  DataStoreName=SSR2  InitialValue=-1  ShowAdditionalParam=off
  Data Store Read : DataStoreRead  DataStoreName=SSR2
  If : If  NumInputs=2  IfExpression=u1 >= a4  ElseIfExpressions=u1 < a1, u2 == -1
  If Action Subsystem1 : Subsystem  TreatAsAtomicUnit=on
  If Action Subsystem2 : Subsystem  TreatAsAtomicUnit=on
  If Action Subsystem3 : Subsystem  TreatAsAtomicUnit=on
  If Action Subsystem4 : Subsystem  TreatAsAtomicUnit=on
  Merge : Merge  Inputs=4
  Mode Acc : Outport
  wires:
  Data Store Read/1 -> If/2
  Constant2/1 -> If Action Subsystem4/1(In1)
  Constant1/1 -> If Action Subsystem3/1(In1)
  W Acc/1 -> If/1
  Merge/1 -> Mode Acc/1
  Constant6/1 -> If Action Subsystem2/1(In1)
  If/4 -> If Action Subsystem3/Action
  If/1 -> If Action Subsystem1/Action
  If Action Subsystem1/1(Out1) -> Merge/1
  If/2 -> If Action Subsystem2/Action
  If Action Subsystem2/1(Out1) -> Merge/2
  Constant/1 -> If Action Subsystem1/1(In1)
  If Action Subsystem4/1(Out1) -> Merge/3
  If Action Subsystem3/1(Out1) -> Merge/4
  If/3 -> If Action Subsystem4/Action

== system CS_ABS_KN_S/KN ABS/FL - L1/Additional Constraint/If Action Subsystem ==
  In1 : Inport
  Action Port : ActionPort  ActionPortLabel=else
  Out1 : Outport
  wires:
  In1/1 -> Out1/1

== system CS_ABS_KN_S/KN ABS/FL - L1/Additional Constraint/If Action Subsystem1 ==
  In1 : Inport
  Action Port : ActionPort  ActionPortLabel=if((u1==1)&(u2<u3))
  Out1 : Outport  InitialOutput=-1
  wires:
  In1/1 -> Out1/1

== system CS_ABS_KN_S/KN ABS/FL - L1/First loop/If Action Subsystem ==
  In1 : Inport
  Action Port : ActionPort  ActionPortLabel=else
  Out1 : Outport
  wires:
  In1/1 -> Out1/1

== system CS_ABS_KN_S/KN ABS/FL - L1/First loop/If Action Subsystem1 ==
  In1 : Inport
  Action Port : ActionPort  ActionPortLabel=if(u1 >= a1)
  Out1 : Outport
  wires:
  In1/1 -> Out1/1

== system CS_ABS_KN_S/KN ABS/FL - L1/First loop/If Action Subsystem2 ==
  In1 : Inport
  Action Port : ActionPort  ActionPortLabel=elseif(u1 < a2)
  Constant1 : Constant  Value=0
  Data Store Write : DataStoreWrite  DataStoreName=FiLoL1
  Out1 : Outport
  wires:
  In1/1 -> Out1/1
  Constant1/1 -> Data Store Write/1

== system CS_ABS_KN_S/KN ABS/FL - L1/Steady State/If Action Subsystem1 ==
  In1 : Inport
  Action Port : ActionPort  ActionPortLabel=if(u1 >= a4)
  Constant : Constant
  Data Store Write : DataStoreWrite  DataStoreName=SSL1
  Out1 : Outport
  wires:
  In1/1 -> Out1/1
  Constant/1 -> Data Store Write/1

== system CS_ABS_KN_S/KN ABS/FL - L1/Steady State/If Action Subsystem2 ==
  In1 : Inport
  Action Port : ActionPort  ActionPortLabel=elseif(u1 < a1)
  Constant : Constant  Value=-1
  Data Store Write : DataStoreWrite  DataStoreName=SSL1
  Out1 : Outport
  wires:
  In1/1 -> Out1/1
  Constant/1 -> Data Store Write/1

== system CS_ABS_KN_S/KN ABS/FL - L1/Steady State/If Action Subsystem3 ==
  In1 : Inport
  Action Port : ActionPort  ActionPortLabel=else
  Out1 : Outport
  wires:
  In1/1 -> Out1/1

== system CS_ABS_KN_S/KN ABS/FL - L1/Steady State/If Action Subsystem4 ==
  In1 : Inport
  Action Port : ActionPort  ActionPortLabel=elseif( u2 == -1)
  Out1 : Outport
  wires:
  In1/1 -> Out1/1

== system CS_ABS_KN_S/KN ABS/FR - R1/Additional Constraint/If Action Subsystem ==
  In1 : Inport
  Action Port : ActionPort  ActionPortLabel=else
  Out1 : Outport
  wires:
  In1/1 -> Out1/1

== system CS_ABS_KN_S/KN ABS/FR - R1/Additional Constraint/If Action Subsystem1 ==
  In1 : Inport
  Action Port : ActionPort  ActionPortLabel=if((u1==1)&(u2<u3))
  Out1 : Outport  InitialOutput=-1
  wires:
  In1/1 -> Out1/1

== system CS_ABS_KN_S/KN ABS/FR - R1/First loop/If Action Subsystem ==
  In1 : Inport
  Action Port : ActionPort  ActionPortLabel=else
  Out1 : Outport
  wires:
  In1/1 -> Out1/1

== system CS_ABS_KN_S/KN ABS/FR - R1/First loop/If Action Subsystem1 ==
  In1 : Inport
  Action Port : ActionPort  ActionPortLabel=if(u1 >= a1)
  Out1 : Outport
  wires:
  In1/1 -> Out1/1

== system CS_ABS_KN_S/KN ABS/FR - R1/First loop/If Action Subsystem2 ==
  In1 : Inport
  Action Port : ActionPort  ActionPortLabel=elseif(u1 < a2)
  Constant1 : Constant  Value=0
  Data Store Write : DataStoreWrite  DataStoreName=FiLoR1
  Out1 : Outport
  wires:
  In1/1 -> Out1/1
  Constant1/1 -> Data Store Write/1

== system CS_ABS_KN_S/KN ABS/FR - R1/Steady State/If Action Subsystem1 ==
  In1 : Inport
  Action Port : ActionPort  ActionPortLabel=if(u1 >= a4)
  Constant : Constant
  Data Store Write : DataStoreWrite  DataStoreName=SSR1
  Out1 : Outport
  wires:
  In1/1 -> Out1/1
  Constant/1 -> Data Store Write/1

== system CS_ABS_KN_S/KN ABS/FR - R1/Steady State/If Action Subsystem2 ==
  In1 : Inport
  Action Port : ActionPort  ActionPortLabel=elseif(u1 < a1)
  Constant : Constant  Value=-1
  Data Store Write : DataStoreWrite  DataStoreName=SSR1
  Out1 : Outport
  wires:
  In1/1 -> Out1/1
  Constant/1 -> Data Store Write/1

== system CS_ABS_KN_S/KN ABS/FR - R1/Steady State/If Action Subsystem3 ==
  In1 : Inport
  Action Port : ActionPort  ActionPortLabel=else
  Out1 : Outport
  wires:
  In1/1 -> Out1/1

== system CS_ABS_KN_S/KN ABS/FR - R1/Steady State/If Action Subsystem4 ==
  In1 : Inport
  Action Port : ActionPort  ActionPortLabel=elseif( u2 == -1)
  Out1 : Outport
  wires:
  In1/1 -> Out1/1

== system CS_ABS_KN_S/KN ABS/RL - L2/Additional Constraint/If Action Subsystem ==
  In1 : Inport
  Action Port : ActionPort  ActionPortLabel=else
  Out1 : Outport
  wires:
  In1/1 -> Out1/1

== system CS_ABS_KN_S/KN ABS/RL - L2/Additional Constraint/If Action Subsystem1 ==
  In1 : Inport
  Action Port : ActionPort  ActionPortLabel=if((u1==1)&(u2<u3))
  Out1 : Outport  InitialOutput=-1
  wires:
  In1/1 -> Out1/1

== system CS_ABS_KN_S/KN ABS/RL - L2/First loop/If Action Subsystem ==
  In1 : Inport
  Action Port : ActionPort  ActionPortLabel=else
  Out1 : Outport
  wires:
  In1/1 -> Out1/1

== system CS_ABS_KN_S/KN ABS/RL - L2/First loop/If Action Subsystem1 ==
  In1 : Inport
  Action Port : ActionPort  ActionPortLabel=if(u1 >= a1)
  Out1 : Outport
  wires:
  In1/1 -> Out1/1

== system CS_ABS_KN_S/KN ABS/RL - L2/First loop/If Action Subsystem2 ==
  In1 : Inport
  Action Port : ActionPort  ActionPortLabel=elseif(u1 < a2)
  Constant1 : Constant  Value=0
  Data Store Write : DataStoreWrite  DataStoreName=FiLoL2
  Out1 : Outport
  wires:
  In1/1 -> Out1/1
  Constant1/1 -> Data Store Write/1

== system CS_ABS_KN_S/KN ABS/RL - L2/Steady State/If Action Subsystem1 ==
  In1 : Inport
  Action Port : ActionPort  ActionPortLabel=if(u1 >= a4)
  Constant : Constant
  Data Store Write : DataStoreWrite  DataStoreName=SSL2
  Out1 : Outport
  wires:
  In1/1 -> Out1/1
  Constant/1 -> Data Store Write/1

== system CS_ABS_KN_S/KN ABS/RL - L2/Steady State/If Action Subsystem2 ==
  In1 : Inport
  Action Port : ActionPort  ActionPortLabel=elseif(u1 < a1)
  Constant : Constant  Value=-1
  Data Store Write : DataStoreWrite  DataStoreName=SSL2
  Out1 : Outport
  wires:
  In1/1 -> Out1/1
  Constant/1 -> Data Store Write/1

== system CS_ABS_KN_S/KN ABS/RL - L2/Steady State/If Action Subsystem3 ==
  In1 : Inport
  Action Port : ActionPort  ActionPortLabel=else
  Out1 : Outport
  wires:
  In1/1 -> Out1/1

== system CS_ABS_KN_S/KN ABS/RL - L2/Steady State/If Action Subsystem4 ==
  In1 : Inport
  Action Port : ActionPort  ActionPortLabel=elseif( u2 == -1)
  Out1 : Outport
  wires:
  In1/1 -> Out1/1

== system CS_ABS_KN_S/KN ABS/RR - R2/Additional Constraint/If Action Subsystem ==
  In1 : Inport
  Action Port : ActionPort  ActionPortLabel=else
  Out1 : Outport
  wires:
  In1/1 -> Out1/1

== system CS_ABS_KN_S/KN ABS/RR - R2/Additional Constraint/If Action Subsystem1 ==
  In1 : Inport
  Action Port : ActionPort  ActionPortLabel=if((u1==1)&(u2<u3))
  Out1 : Outport  InitialOutput=-1
  wires:
  In1/1 -> Out1/1

== system CS_ABS_KN_S/KN ABS/RR - R2/First loop/If Action Subsystem ==
  In1 : Inport
  Action Port : ActionPort  ActionPortLabel=else
  Out1 : Outport
  wires:
  In1/1 -> Out1/1

== system CS_ABS_KN_S/KN ABS/RR - R2/First loop/If Action Subsystem1 ==
  In1 : Inport
  Action Port : ActionPort  ActionPortLabel=if(u1 >= a1)
  Out1 : Outport
  wires:
  In1/1 -> Out1/1

== system CS_ABS_KN_S/KN ABS/RR - R2/First loop/If Action Subsystem2 ==
  In1 : Inport
  Action Port : ActionPort  ActionPortLabel=elseif(u1 < a2)
  Constant1 : Constant  Value=0
  Data Store Write : DataStoreWrite  DataStoreName=FiLoR2
  Out1 : Outport
  wires:
  In1/1 -> Out1/1
  Constant1/1 -> Data Store Write/1

== system CS_ABS_KN_S/KN ABS/RR - R2/Steady State/If Action Subsystem1 ==
  In1 : Inport
  Action Port : ActionPort  ActionPortLabel=if(u1 >= a4)
  Constant : Constant
  Data Store Write : DataStoreWrite  DataStoreName=SSR2
  Out1 : Outport
  wires:
  In1/1 -> Out1/1
  Constant/1 -> Data Store Write/1

== system CS_ABS_KN_S/KN ABS/RR - R2/Steady State/If Action Subsystem2 ==
  In1 : Inport
  Action Port : ActionPort  ActionPortLabel=elseif(u1 < a1)
  Constant : Constant  Value=-1
  Data Store Write : DataStoreWrite  DataStoreName=SSR2
  Out1 : Outport
  wires:
  In1/1 -> Out1/1
  Constant/1 -> Data Store Write/1

== system CS_ABS_KN_S/KN ABS/RR - R2/Steady State/If Action Subsystem3 ==
  In1 : Inport
  Action Port : ActionPort  ActionPortLabel=else
  Out1 : Outport
  wires:
  In1/1 -> Out1/1

== system CS_ABS_KN_S/KN ABS/RR - R2/Steady State/If Action Subsystem4 ==
  In1 : Inport
  Action Port : ActionPort  ActionPortLabel=elseif( u2 == -1)
  Out1 : Outport
  wires:
  In1/1 -> Out1/1
